simulink model "simulationScheme"  (R2021a)
settings: Solver=VariableStepAuto  StartTime=0.0  StopTime=7  RelTol=1e-3
values from neighbouring files (symbols this model uses):
  C = [ 1   0   0   0; 0   0   1   0]    [lpvGainScheduled.m]    (also in main.m = [1 0 0 0;0 1 0 0;0 0 1 0;0 0 0 1])
  Car = 80000    [main.m]
  K = W / X    [controlloreDstabilita.m]    (also in controlloreH2.m; controlloreHinfinito.m; controlloreL1.m; controlloreRobustoH2.m)
  Kv = ((lr*m)/(2*Caf*L))-((lf*m)/(2*Car*L))    (= 0.00176082089552)    [main.m]
  L = lf+lr    (= 2.68)    [main.m]
  lf = 1.1    [main.m]
  lr = 1.58    [main.m]
  m = 10.8    [lpvGainScheduled.m]    (also in main.m = 1573)
  Ts = 0.01    [lpvGainScheduled.m]    (also in main.m)
  Vx = 30    [main.m]
libraries: drivingscenarioandsensors x1, autolibshared x1
settings Model: EnablePacing=on  PacingRate=0.710000  Creator=nicol  LastModifiedBy=nicol

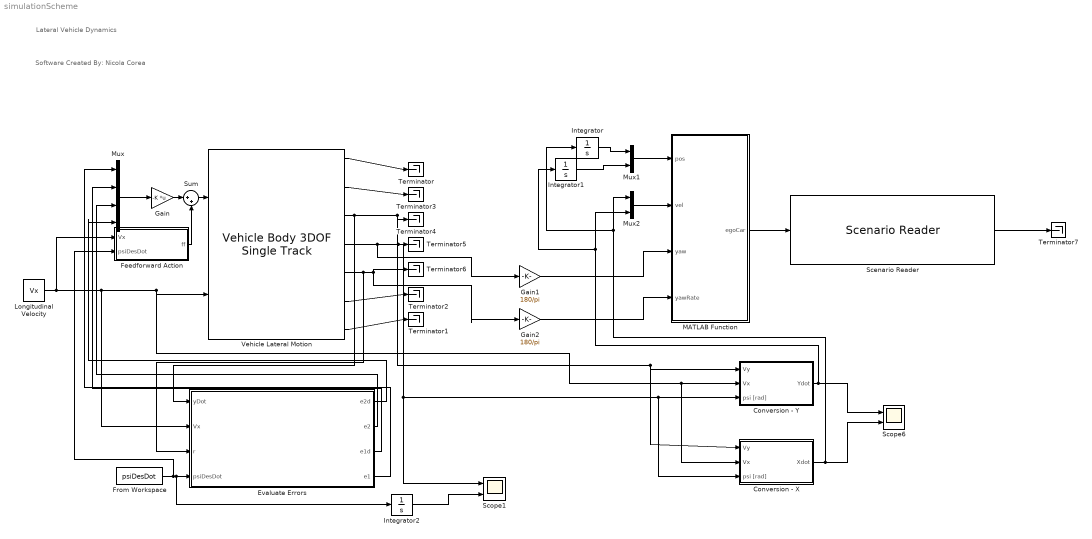
== system simulationScheme ==
  note: Software Created By: Nicola Corea
  note: Lateral Vehicle Dynamics
  Conversion - X : Subsystem
  Conversion - Y : Subsystem
  Evaluate Errors : Subsystem
  Feedforward Action : Subsystem
  From Workspace : FromWorkspace  VariableName=psiDesDot
  Gain : Gain  Gain=-K  Multiplication=Matrix(K*u) (u vector)
  Gain1 : Gain  Gain=180/pi
  Gain2 : Gain  Gain=180/pi
  Integrator : Integrator  InitialCondition=-51.60
  Integrator1 : Integrator  InitialCondition=-45.30
  Integrator2 : Integrator
  Longitudinal Velocity : Constant  Value=Vx
  MATLAB Function : MATLAB Function  TreatAsAtomicUnit=on
  Mux : Mux
  Mux1 : Mux  Inputs=2
  Mux2 : Mux  Inputs=2
  Scenario Reader : drivingscenarioandsensors/Scenario Reader  ScenarioSource=From file  ScenarioFileName=C:\Users\nicol\Desktop\DrivingScenarioLateral\simulationScenario.mat  ScenarioVariableName=scenario  OutputCoordinateSystem=Vehicle coordinates  EgoVehicleSource=Input port  EgoVehicleActorID=1  OrientVehiclesOnRoad=on  OutputEgoVehiclePose=off  SampleTime=Ts  LaneBoundaryOutput=None  LaneBoundaryDistance=0:0.5:9.5  LaneBoundaryLocation=Center of lane markings  BusNameSource=Auto  BusName=BusActors  BusNumActorsSource=Scenario  BusNumActors=100  BusName2Source=Auto  BusName2=BusLaneBoundaries  BusNumLaneBoundariesSource=Scenario  BusNumLaneBoundaries=10  BusName3Source=Auto  BusName3=BusEgoActor  ShowCoordinateLabels=on  SimulateUsing=Interpreted execution
  Scope1 : Scope  NumInputPorts=2
  Scope6 : Scope  NumInputPorts=2
  Sum : Sum  Inputs=|++
  Terminator{,1..7} (8 alike) : Terminator
  Vehicle Lateral Motion : autolibshared/Vehicle Body 3DOF Single Track  trackMode=Single (bicycle)  inputMode=External longitudinal velocity  frontSteerMode=on  rearSteerMode=off  windMode=off  muMode=off  extFMode=off  extMMode=off  htchFMode=off  htchMMode=off  extXo=off  extpsio=off  extxdoto=off  extro=off  extYo=off  extTamb=off  extydoto=off  aMode=2  NF=2  NR=2  m=m  a=lf  b=lr  h=0.35  dh=1  hh=0.2  X_o=0  xdot_o=0  CalphaMode=off  sigmaMode=on  d=0  hl=0  w=[1.4,1.4]  Cy_f=Caf  Cy_r=Car  sigma_f=.1  sigma_r=.1  alpha_f_brk=[-.1 .1]  Cy_f_data=[-9e3 9e3]  alpha_r_brk=[-.1 .1]  Cy_r_data=[-9e3 9e3]  Y_o=0  ydot_o=0  Izz=Iz  psi_o=0  r_o=0  Af=2  Cd=.3  Cl=.1  Cpm=.1  beta_w=[0:0.01:0.3]  Cs=[0:0.03:0.9]  Cym=[0:0.01:0.3]  Pabs=101325  Tair=273  g=9.81  mu=1  xdot_tol=.01  Fznom=5000  Fxtire_sat=7e4  Fytire_sat=7e4  longOff=0  latOff=0  vertOff=0  wrapAng=off
      settings: SourceProductBaseCode=PW,DR,MT,UV,VE
  wires:
  Longitudinal Velocity/1 -> Feedforward Action/1(Vx), Evaluate Errors/2(Vx), Conversion - X/2(Vx), Conversion - Y/2(Vx), Vehicle Lateral Motion/2
  Vehicle Lateral Motion/1 -> Terminator/1
  Vehicle Lateral Motion/7 -> Terminator1/1
  Vehicle Lateral Motion/6 -> Terminator2/1
  Vehicle Lateral Motion/5 -> Evaluate Errors/3(r), Gain2/1, Terminator6/1
  Vehicle Lateral Motion/4 -> Gain1/1, Scope1/1, Conversion - X/3(psi [rad]), Conversion - Y/3(psi [rad]), Terminator5/1
  Vehicle Lateral Motion/3 -> Evaluate Errors/1(yDot), Conversion - X/1(Vy), Conversion - Y/1(Vy), Terminator4/1
  Vehicle Lateral Motion/2 -> Terminator3/1
  From Workspace/1 -> Feedforward Action/2(psiDesDot), Integrator2/1, Evaluate Errors/4(psiDesDot)
  Evaluate Errors/4(e1) -> Mux/1
  Evaluate Errors/3(e1d) -> Mux/2
  Evaluate Errors/2(e2) -> Mux/3
  Evaluate Errors/1(e2d) -> Mux/4
  Mux/1 -> Gain/1
  Scenario Reader/1 -> Terminator7/1
  MATLAB Function/1(egoCar) -> Scenario Reader/1
  Mux1/1 -> MATLAB Function/1(pos)
  Mux2/1 -> MATLAB Function/2(vel)
  Conversion - X/1(Xdot) -> Integrator/1, Mux2/1, Scope6/2
  Integrator/1 -> Mux1/1
  Integrator1/1 -> Mux1/2
  Conversion - Y/1(Ydot) -> Integrator1/1, Mux2/2, Scope6/1
  Gain1/1 -> MATLAB Function/3(yaw)
  Gain2/1 -> MATLAB Function/4(yawRate)
  Gain/1 -> Sum/1
  Sum/1 -> Vehicle Lateral Motion/1
  Feedforward Action/1(ff) -> Sum/2
  Integrator2/1 -> Scope1/2

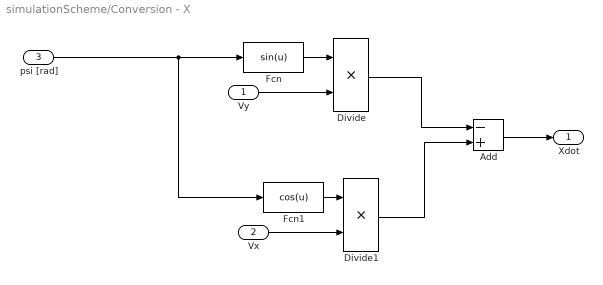
== system simulationScheme/Conversion - X ==
  Vy : Inport
  Vx : Inport  Port=2
  psi [rad] : Inport  Port=3
  Add : Sum  Inputs=-+
  Divide : Product  Inputs=**
  Divide1 : Product  Inputs=**
  Fcn : Fcn  Expr=sin(u)
  Fcn1 : Fcn  Expr=cos(u)
  Xdot : Outport
  wires:
  psi [rad]/1 -> Fcn/1, Fcn1/1
  Add/1 -> Xdot/1
  Divide1/1 -> Add/2
  Vx/1 -> Divide1/2
  Fcn1/1 -> Divide1/1
  Divide/1 -> Add/1
  Vy/1 -> Divide/2
  Fcn/1 -> Divide/1

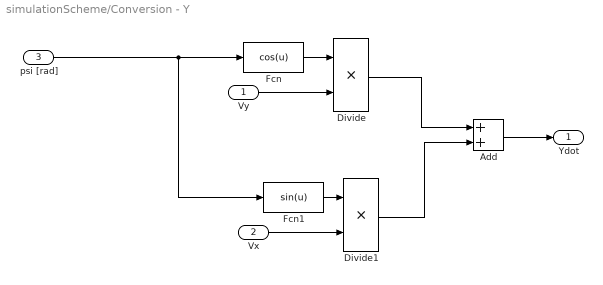
== system simulationScheme/Conversion - Y ==
  Vy : Inport
  Vx : Inport  Port=2
  psi [rad] : Inport  Port=3
  Add : Sum
  Divide : Product  Inputs=**
  Divide1 : Product  Inputs=**
  Fcn : Fcn  Expr=cos(u)
  Fcn1 : Fcn  Expr=sin(u)
  Ydot : Outport
  wires:
  Fcn/1 -> Divide/1
  Vy/1 -> Divide/2
  Divide/1 -> Add/1
  Fcn1/1 -> Divide1/1
  Vx/1 -> Divide1/2
  Divide1/1 -> Add/2
  Add/1 -> Ydot/1
  psi [rad]/1 -> Fcn1/1, Fcn/1

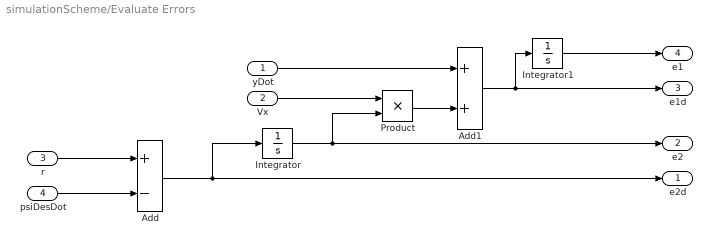
== system simulationScheme/Evaluate Errors ==
  yDot : Inport
  Vx : Inport  Port=2
  r : Inport  Port=3
  psiDesDot : Inport  Port=4
  Add : Sum  Inputs=+-
  Add1 : Sum
  Integrator : Integrator
  Integrator1 : Integrator
  Product : Product
  e2d : Outport
  e2 : Outport  Port=2
  e1d : Outport  Port=3
  e1 : Outport  Port=4
  wires:
  Product/1 -> Add1/2
  Integrator/1 -> e2/1, Product/2
  Add1/1 -> e1d/1, Integrator1/1
  Vx/1 -> Product/1
  Add/1 -> e2d/1, Integrator/1
  Integrator1/1 -> e1/1
  r/1 -> Add/1
  yDot/1 -> Add1/1
  psiDesDot/1 -> Add/2

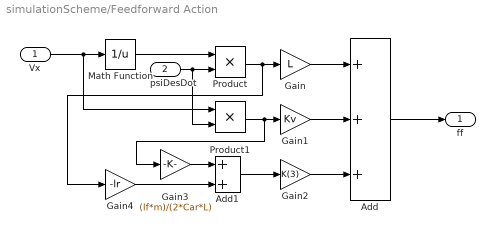
== system simulationScheme/Feedforward Action ==
  Vx : Inport
  psiDesDot : Inport  Port=2
  Add : Sum  Inputs=+++
  Add1 : Sum
  Gain : Gain  Gain=L
  Gain1 : Gain  Gain=Kv
  Gain2 : Gain  Gain=K(3)
  Gain3 : Gain  Gain=(lf*m)/(2*Car*L)
  Gain4 : Gain  Gain=-lr
  Math Function : Math  Operator=reciprocal  SaturateOnIntegerOverflow=on
  Product : Product
  Product1 : Product
  ff : Outport
  wires:
  Add/1 -> ff/1
  Gain/1 -> Add/1
  Product/1 -> Gain4/1, Gain/1
  Math Function/1 -> Product/1
  Vx/1 -> Product1/1, Math Function/1
  psiDesDot/1 -> Product1/2, Product/2
  Gain1/1 -> Add/2
  Product1/1 -> Gain3/1, Gain1/1
  Gain2/1 -> Add/3
  Add1/1 -> Gain2/1
  Gain3/1 -> Add1/1
  Gain4/1 -> Add1/2

== matlab function simulationScheme/MATLAB Function ==
  data: pos input; egoCar output Bus: BusActors1Actors; vel input; yaw input; yawRate input
function egoCar = packEgo(pos,vel,yaw,yawRate)
egoCar = struct('ActorID',1,...
                'Position',[pos(1) pos(2) 0],...
                'Velocity',[vel(1) vel(2) 0],...
                'Roll',0,...
                'Pitch',0,...
                'Yaw',yaw,...
                'AngularVelocity',[0 0 yawRate]);
end
